simulink model "parameters_const"  (R2023b)
settings: Solver=ode3  StartTime=0.0  StopTime=Tmdl  FixedStep=1e-4  MaxStep=0.001  RelTol=1e-3
undefined symbols (not defined in the file): J, K1, K2, K3, K4, Ki, Ku, Lm, Lr, Mn, Mn_coef, Mn_flag, zp
settings Model: Creator=ver0sunny  LastModifiedBy=deniskirbaba
settings ModelReferenceCC: EnableRefExpFcnMdlSchedulingChecks=on

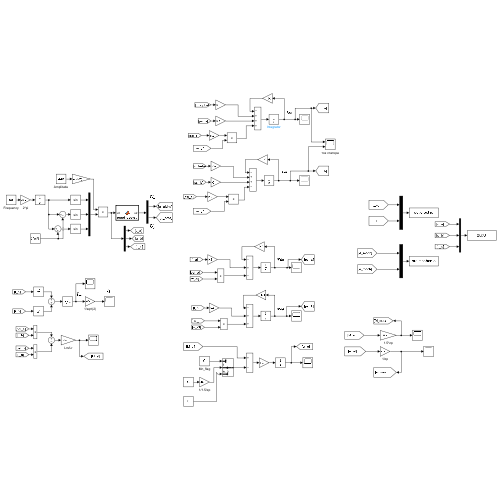
[thumbnail: Simulink's stored preview of the top-level diagram]
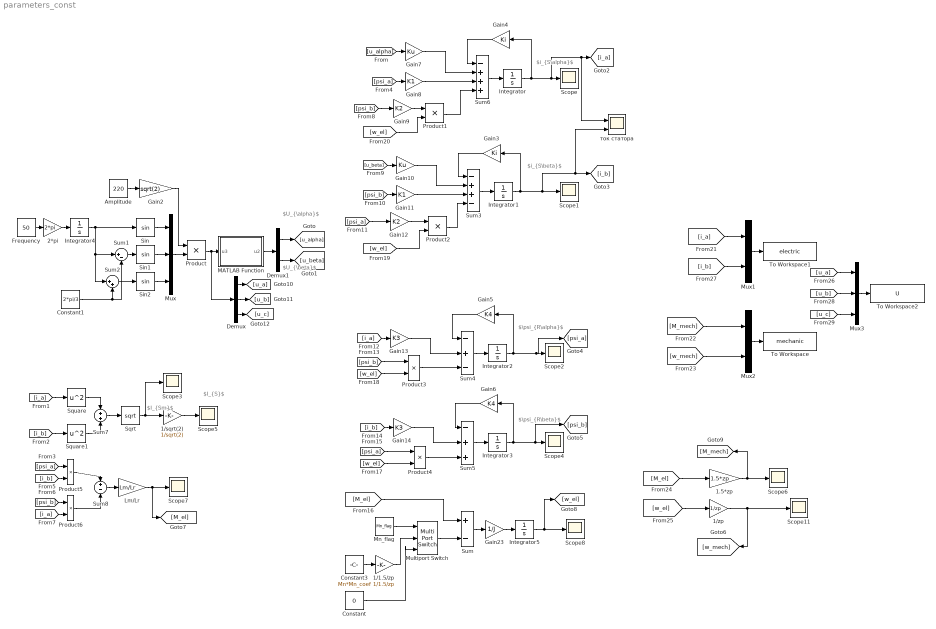
== system parameters_const ==
  note: $U_{\alpha}$
  note: $U_{\beta}$
  note: $i_{S\alpha}$
  note: $i_{S\beta}$
  note: $\psi_{R\alpha}$
  note: $\psi_{R\beta}$
  note: $I_{S}$
  note: $I_{Sm}$
  1.5*zp : Gain  Gain=1.5*zp
  1/1.5/zp : Gain  Gain=1/1.5/zp
  1/sqrt(2) : Gain  Gain=1/sqrt(2)
  1/zp : Gain  Gain=1/zp
  2*pi : Gain  Gain=2*pi
  Amplitude : Constant  Value=220
  Constant : Constant  Value=0
  Constant1 : Constant  Value=2*pi/3
  Constant3 : Constant  Value=Mn*Mn_coef
  Demux : Demux  Outputs=3
  Demux1 : Demux  Outputs=2
  Frequency : Constant  Value=50
  Gain10 : Gain  Gain=Ku
  Gain11 : Gain  Gain=K1
  Gain12 : Gain  Gain=K2
  Gain13 : Gain  Gain=K3
  Gain14 : Gain  Gain=K3
  Gain2 : Gain  Gain=sqrt(2)
  Gain23 : Gain  Gain=1/J
  Gain3 : Gain  Gain=Ki
  Gain4 : Gain  Gain=Ki
  Gain5 : Gain  Gain=K4
  Gain6 : Gain  Gain=K4
  Gain7 : Gain  Gain=Ku
  Gain8 : Gain  Gain=K1
  Gain9 : Gain  Gain=K2
  Integrator{,1..5} (6 alike) : Integrator
  Lm/Lr : Gain  Gain=Lm/Lr
  MATLAB Function : MATLAB Function  TreatAsAtomicUnit=on
  Mn_flag : Constant  Value=Mn_flag
  Multiport Switch : MultiPortSwitch  Inputs=2  SaturateOnIntegerOverflow=off  InputSameDT=off
  Mux : Mux  Inputs=3
  Mux1 : Mux  Inputs=2
  Mux2 : Mux  Inputs=2
  Mux3 : Mux  Inputs=3
  Product{,1..6} (7 alike) : Product
  Scope{,1..8,11} (10 alike) : Scope
  Sin : Trigonometry
  Sin1 : Trigonometry
  Sin2 : Trigonometry
  Sqrt : Sqrt
  Square : Math  Operator=square
  Square1 : Math  Operator=square
  Sum : Sum  Inputs=+-
  Sum1 : Sum  Inputs=|+-
  Sum2 : Sum  Inputs=|++
  Sum3 : Sum  Inputs=-++-
  Sum4 : Sum  Inputs=-+-
  Sum5 : Sum  Inputs=-++
  Sum6 : Sum  Inputs=-+++
  Sum7 : Sum  Inputs=+|+
  Sum8 : Sum  Inputs=+|-
  To Workspace : ToWorkspace  VariableName=mechanic  SaveFormat=Timeseries  SampleTime=-1
  To Workspace1 : ToWorkspace  VariableName=electric  SaveFormat=Timeseries  SampleTime=-1
  To Workspace2 : ToWorkspace  VariableName=U  SaveFormat=Timeseries  SampleTime=-1
  ток статора : Scope  NumInputPorts=2
  wires:
  Integrator/1 -> ток статора/1, [i_a], Scope/1, Gain4/1
  Frequency/1 -> 2*pi/1
  Sin2/1 -> Mux/3
  Sin1/1 -> Mux/2
  Integrator4/1 -> Sum1/1, Sum2/1, Sin/1
  Sin/1 -> Mux/1
  Gain2/1 -> Product/1
  Mux/1 -> Product/2
  Sum2/1 -> Sin2/1
  Sum1/1 -> Sin1/1
  2*pi/1 -> Integrator4/1
  Constant1/1 -> Sum1/2, Sum2/2
  Amplitude/1 -> Gain2/1
  Product/1 -> Demux/1, MATLAB Function/1(u3)
  MATLAB Function/1(u2) -> Demux1/1
  Demux1/1 -> [u_alpha]
  Demux1/2 -> [u_beta]
  Sum3/1 -> Integrator1/1
  Sum4/1 -> Integrator2/1
  Sum5/1 -> Integrator3/1
  Sum6/1 -> Integrator/1
  Gain4/1 -> Sum6/1
  Gain3/1 -> Sum3/1
  Integrator2/1 -> Gain5/1, [psi_a], Scope2/1
  Gain5/1 -> Sum4/1
  Integrator3/1 -> Gain6/1, [psi_b], Scope4/1
  Gain6/1 -> Sum5/1
  [u_alpha] -> Gain7/1
  Gain7/1 -> Sum6/2
  [psi_a] -> Gain8/1
  Gain8/1 -> Sum6/3
  [psi_b] -> Gain9/1
  [psi_a] -> Gain12/1
  Gain11/1 -> Sum3/3
  [psi_b] -> Gain11/1
  Gain10/1 -> Sum3/2
  [u_beta] -> Gain10/1
  [i_a] -> Gain13/1
  Gain13/1 -> Sum4/2
  [psi_b] -> Product3/1
  [psi_a] -> Product4/1
  Gain14/1 -> Sum5/2
  [i_b] -> Gain14/1
  Square1/1 -> Sum7/2
  Sum7/1 -> Sqrt/1
  Square/1 -> Sum7/1
  1/sqrt(2)/1 -> Scope5/1
  Sqrt/1 -> Scope3/1, 1/sqrt(2)/1
  [i_a] -> Square/1
  [i_b] -> Square1/1
  [i_b] -> Product5/2
  [psi_a] -> Product5/1
  Product5/1 -> Sum8/1
  [psi_b] -> Product6/1
  [i_a] -> Product6/2
  Product6/1 -> Sum8/2
  Sum8/1 -> Lm/Lr/1
  Product3/1 -> Sum4/3
  [M_el] -> Sum/1
  Sum/1 -> Gain23/1
  Gain23/1 -> Integrator5/1
  Integrator5/1 -> [w_el], Scope8/1
  Gain9/1 -> Product1/1
  Product1/1 -> Sum6/4
  Gain12/1 -> Product2/1
  Product2/1 -> Sum3/4
  Product4/1 -> Sum5/3
  [w_el] -> Product1/2
  [w_el] -> Product2/2
  [w_el] -> Product3/2
  [w_el] -> Product4/2
  Lm/Lr/1 -> [M_el], Scope7/1
  Integrator1/1 -> Gain3/1, ток статора/2, [i_b], Scope1/1
  [M_mech] -> Mux2/1
  [w_mech] -> Mux2/2
  Mux2/1 -> To Workspace/1
  [w_el] -> 1/zp/1
  1.5*zp/1 -> Scope6/1, [M_mech]
  [M_el] -> 1.5*zp/1
  1/zp/1 -> Scope11/1, [w_mech]
  Constant3/1 -> 1/1.5/zp/1
  Mux1/1 -> To Workspace1/1
  [i_a] -> Mux1/1
  [i_b] -> Mux1/2
  Demux/1 -> [u_a]
  Demux/2 -> [u_b]
  Demux/3 -> [u_c]
  [u_a] -> Mux3/1
  Mux3/1 -> To Workspace2/1
  [u_b] -> Mux3/2
  [u_c] -> Mux3/3
  Multiport Switch/1 -> Sum/2
  1/1.5/zp/1 -> Multiport Switch/2
  Constant/1 -> Multiport Switch/3
  Mn_flag/1 -> Multiport Switch/1

== matlab function parameters_const/MATLAB Function ==
  data: u3 input; u2 output
function u2 = preobrazovat(u3)
    u2 = [2/3 -(1/3) -(1/3); 0 1/sqrt(3) -1/sqrt(3)] * u3;
end
